simulink model "PidDiscrete"  (R2024b)
settings: Solver=VariableStepAuto  StartTime=0.0  StopTime=10.0  RelTol=1e-3
values from neighbouring files (symbols this model uses):
  Hd = tf(numd, dend, 1/fs)    [modeling.m]
undefined symbols (not defined in the file or in its folder): DiscIntNeverNeededParam, Kd, Ki, Kp
libraries: simulink x1
settings Model: Creator=bolinsfe  LastModifiedBy=bolinsfe

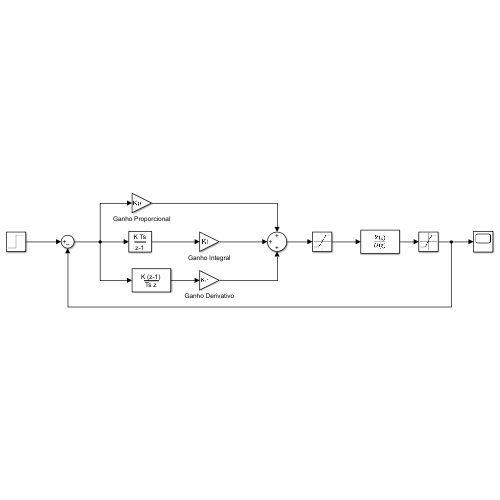
[thumbnail: Simulink's stored preview of the top-level diagram]
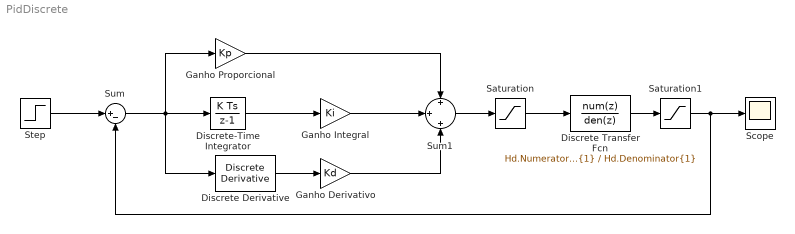
== system PidDiscrete ==
  Discrete Transfer Fcn : DiscreteTransferFcn  Numerator=Hd.Numerator{1}  Denominator=Hd.Denominator{1}
  Discrete Derivative : simulink/Discrete/Discrete Derivative  gainval=1.0  ICPrevScaledInput=0.0  OutMin=[]  OutMax=[]  OutDataType=fixdt(1, 16)  OutScaling=2^-10  DoSatur=off
  Discrete-Time Integrator : DiscreteIntegrator  SampleTime=0.02  ICPrevOutput=DiscIntNeverNeededParam  ICPrevScaledInput=DiscIntNeverNeededParam
  Ganho Derivativo : Gain  Gain=Kd
  Ganho Integral : Gain  Gain=Ki
  Ganho Proporcional : Gain  Gain=Kp
  Saturation : Saturate  UpperLimit=30  LowerLimit=-30
  Saturation1 : Saturate  UpperLimit=80  LowerLimit=0
  Scope : Scope
  Step : Step  Time=0.010  After=20  SampleTime=0
  Sum : Sum  Inputs=|+-
  Sum1 : Sum  Inputs=+|+|+
  wires:
  Ganho Integral/1 -> Sum1/2
  Ganho Proporcional/1 -> Sum1/1
  Step/1 -> Sum/1
  Discrete Derivative/1 -> Ganho Derivativo/1
  Sum1/1 -> Saturation/1
  Ganho Derivativo/1 -> Sum1/3
  Sum/1 -> Discrete-Time Integrator/1, Discrete Derivative/1, Ganho Proporcional/1
  Discrete-Time Integrator/1 -> Ganho Integral/1
  Saturation/1 -> Discrete Transfer Fcn/1
  Discrete Transfer Fcn/1 -> Saturation1/1
  Saturation1/1 -> Sum/2, Scope/1
